simulink model "Winda4"  (R2016a)
settings: Solver=FixedStepDiscrete  StartTime=0.0  StopTime=inf  FixedStep=0.05  MaxStep=0.1  MinStep=0.01  RelTol=1e-3
libraries: simulink x15, realtime_pacer_lib x2
settings Model: Creator=dmar  LastModifiedBy=Kuba
settings DataIOCC: LimitDataPoints=on  SaveFormat=Array  SignalLoggingSaveFormat=ModelDataLogs  SignalLogging=off
settings OptimizationCC: BlockReduction=off  ConditionallyExecuteInputs=off  ExpressionDepthLimit=2147483647
settings DebuggingCC: AlgebraicLoopMsg=error  UnderspecifiedInitializationDetection=Classic  MergeDetectMultiDrivingBlocksExec=none  SolverPrmCheckMsg=warning  ParameterPrecisionLossMsg=none  FcnCallInpInsideContextMsg=UseLocalSettings  AllowSymbolicDim=off  StateNameClashWarn=warning
settings HardwareCC: ProdBitPerPointer=32  ProdLargestAtomicFloat=None  ProdIntDivRoundTo=Undefined  ProdEndianess=Unspecified  ProdWordSize=32  ProdHWDeviceType=ASIC/FPGA->ASIC/FPGA  ProdEqTarget=off
settings ModelReferenceCC: PropagateSignalLabelsOutOfModel=off
settings SFSimCC: SimParseCustomCode=off
settings GRTTargetCC: CombineOutputUpdateFcns=off  GRTInterface=on
settings ConfigComp: CovModelRefEnable=Off

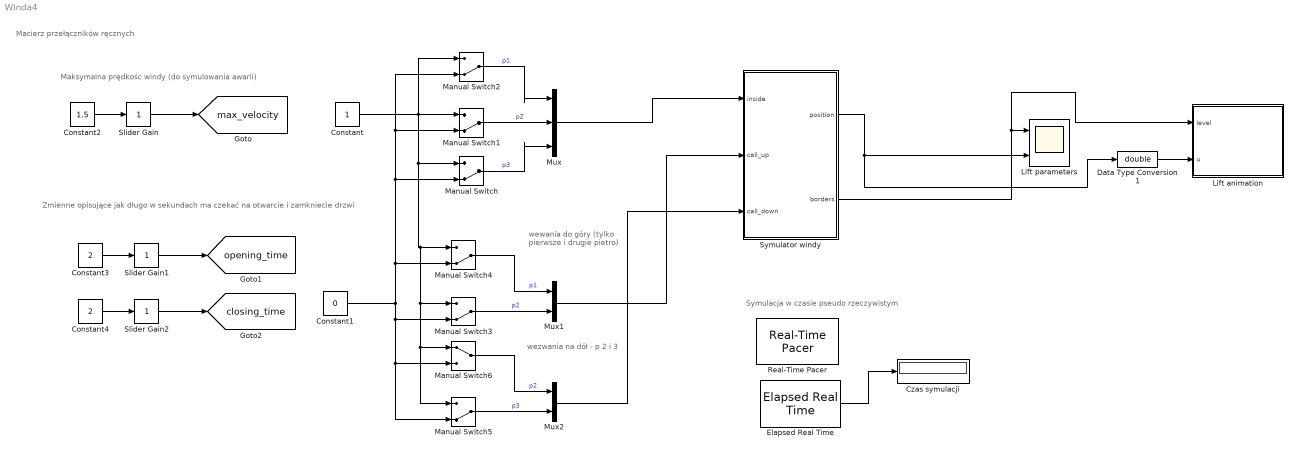
== system Winda4 ==
  note: wezwania na dół - p 2 i 3
  note: wewania do góry
      | (tylko pierwsze i drugie
      | pietro)
  note: Zmienne opisujące jak długo w sekundach ma czekać na otwarcie i zamkniecie drzwi
  note: Maksymalna prędkośc windy (do symulowania awarii)
  note: Macierz przełączników ręcznych
  note: Symulacja w czasie pseudo rzeczywistym
  Constant : Constant
  Constant1 : Constant  Value=0
  Constant2 : Constant  Value=1.5
  Constant3 : Constant  Value=2
  Constant4 : Constant  Value=2
  Czas symulacji : Display
  Data Type Conversion1 : DataTypeConversion  OutDataTypeStr=double
  Elapsed Real Time : realtime_pacer_lib/Elapsed Real Time
  Lift animation : MATLAB Function  TreatAsAtomicUnit=on  SystemSampleTime=0.05
  Lift parameters : Scope  NumInputPorts=2
  Manual Switch{,1..5} (6 alike) : ManualSwitch  CurrentSetting=0
  Manual Switch6 : ManualSwitch
  Mux : Mux  Inputs=3
  Mux1 : Mux  Inputs=2
  Mux2 : Mux  Inputs=2
  Real-Time Pacer : realtime_pacer_lib/Real-Time Pacer  simTimePerRealTime=1
  Slider Gain : simulink/Math Operations/Slider Gain  low=0  gain=1  high=1
  Slider Gain1 : simulink/Math Operations/Slider Gain  low=0  gain=1  high=1
  Slider Gain2 : simulink/Math Operations/Slider Gain  low=0  gain=1  high=1
  Symulator windy : Subsystem
  tag scope: closing_time=global, max_velocity=global, opening_time=global
  wires:
  Data Type Conversion1/1 -> Lift animation/2(u)
  Symulator windy/1(position) -> Data Type Conversion1/1, Lift parameters/2
  Symulator windy/2(borders) -> Lift animation/1(level), Lift parameters/1
  Elapsed Real Time/1 -> Czas symulacji/1
  Mux/1 -> Symulator windy/1(inside)
  Mux1/1 -> Symulator windy/2(call_up)
  Mux2/1 -> Symulator windy/3(call_down)
  Manual Switch6/1 -> Mux2/1  "p2"
  Constant/1 -> Manual Switch2/1, Manual Switch6/1, Manual Switch5/1, Manual Switch3/1, Manual Switch4/1, Manual Switch/1, Manual Switch1/1
  Constant1/1 -> Manual Switch2/2, Manual Switch1/2, Manual Switch/2, Manual Switch4/2, Manual Switch5/2, Manual Switch6/2, Manual Switch3/2
  Manual Switch5/1 -> Mux2/2  "p3"
  Manual Switch3/1 -> Mux1/2  "p2"
  Manual Switch4/1 -> Mux1/1  "p1"
  Manual Switch1/1 -> Mux/2  "p2"
  Manual Switch/1 -> Mux/3  "p3"
  Manual Switch2/1 -> Mux/1  "p1"
  Constant2/1 -> Slider Gain/1
  Slider Gain/1 -> [max_velocity]
  Constant3/1 -> Slider Gain1/1
  Slider Gain1/1 -> [opening_time]
  Constant4/1 -> Slider Gain2/1
  Slider Gain2/1 -> [closing_time]

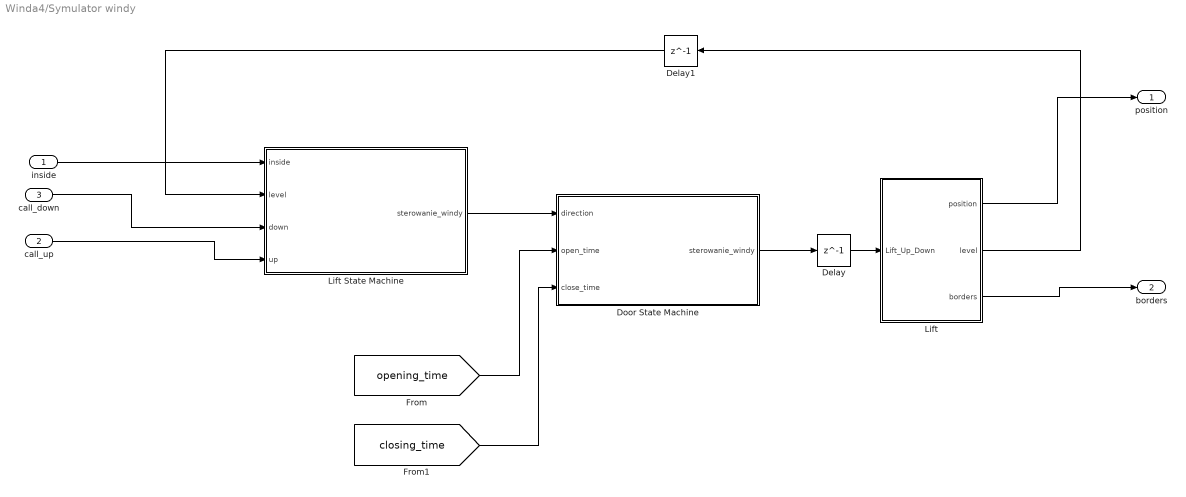
== system Winda4/Symulator windy ==
  inside : Inport
  call_up : Inport  Port=2
  call_down : Inport  Port=3
  Delay : Delay  DelayLength=1  InitialCondition=0
  Delay1 : Delay  DelayLength=1  InitialCondition=0
  Door State Machine : Stateflow chart  TreatAsAtomicUnit=on
  Lift : Subsystem
  Lift State Machine : Stateflow chart  TreatAsAtomicUnit=on
  position : Outport
  borders : Outport  Port=2
  wires:
  Lift/1(position) -> position/1
  Delay/1 -> Lift/1(Lift_Up_Down)
  inside/1 -> Lift State Machine/1(inside)
  Lift/2(level) -> Delay1/1
  Lift/3(borders) -> borders/1
  Delay1/1 -> Lift State Machine/2(level)
  Door State Machine/1(sterowanie_windy) -> Delay/1
  Lift State Machine/1(sterowanie_windy) -> Door State Machine/1(direction)
  call_down/1 -> Lift State Machine/3(down)
  call_up/1 -> Lift State Machine/4(up)
  [opening_time] -> Door State Machine/2(open_time)
  [closing_time] -> Door State Machine/3(close_time)

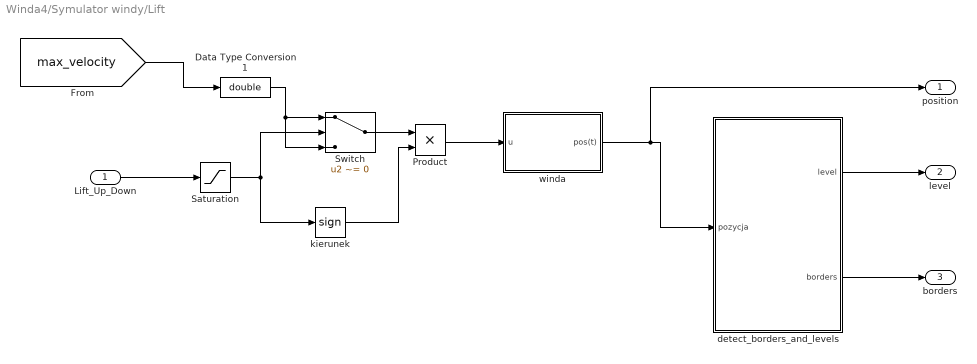
== system Winda4/Symulator windy/Lift ==
  Lift_Up_Down : Inport  OutDataTypeStr=int8
  Data Type Conversion1 : DataTypeConversion  OutDataTypeStr=double
  Product : Product  OutDataTypeStr=Inherit: Inherit via back propagation  RndMeth=Zero
  Saturation : Saturate  UpperLimit=1  LowerLimit=-1
  Switch : Switch  Criteria=u2 ~= 0  OutDataTypeStr=Inherit: Inherit via back propagation
  detect_borders_and_levels : Subsystem
  kierunek : Signum
  winda : Subsystem
  position : Outport
  level : Outport  Port=2
  borders : Outport  Port=3
  wires:
  Lift_Up_Down/1 -> Saturation/1
  Switch/1 -> Product/1
  Product/1 -> winda/1(u)
  kierunek/1 -> Product/2
  winda/1(pos(t)) -> detect_borders_and_levels/1(pozycja), position/1
  Saturation/1 -> Switch/2, kierunek/1
  detect_borders_and_levels/1(level) -> level/1
  detect_borders_and_levels/2(borders) -> borders/1
  [max_velocity] -> Data Type Conversion1/1
  Data Type Conversion1/1 -> Switch/3, Switch/1

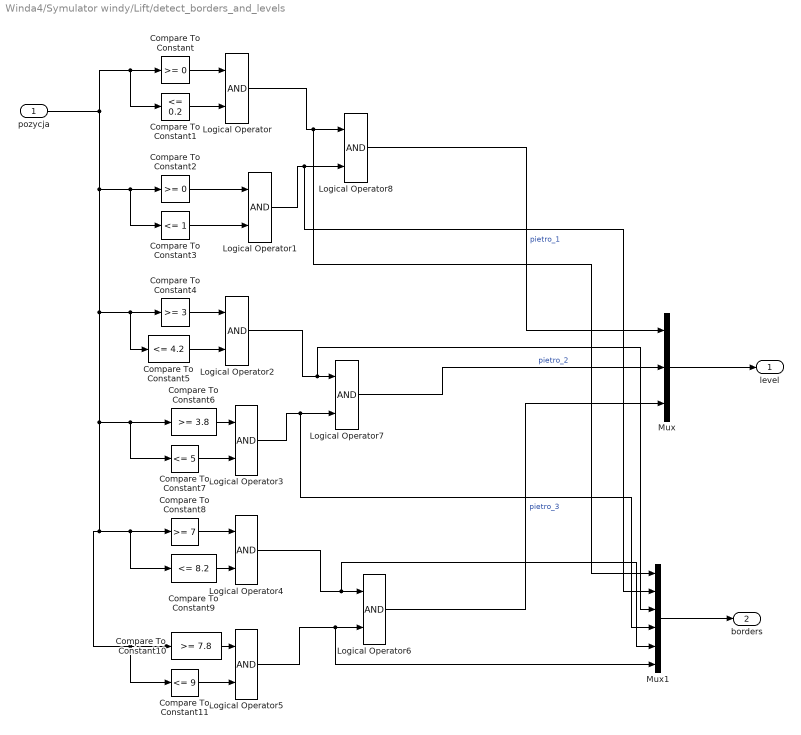
== system Winda4/Symulator windy/Lift/detect_borders_and_levels ==
  pozycja : Inport
  Compare To Constant : simulink/Logic and Bit Operations/Compare To Constant  relop=>=  const=0  OutDataTypeStr=boolean
  Compare To Constant1 : simulink/Logic and Bit Operations/Compare To Constant  relop=<=  const=0.2  OutDataTypeStr=boolean
  Compare To Constant10 : simulink/Logic and Bit Operations/Compare To Constant  relop=>=  const=7.8  OutDataTypeStr=boolean
  Compare To Constant11 : simulink/Logic and Bit Operations/Compare To Constant  relop=<=  const=9  OutDataTypeStr=boolean
  Compare To Constant2 : simulink/Logic and Bit Operations/Compare To Constant  relop=>=  const=0  OutDataTypeStr=boolean
  Compare To Constant3 : simulink/Logic and Bit Operations/Compare To Constant  relop=<=  const=1  OutDataTypeStr=boolean
  Compare To Constant4 : simulink/Logic and Bit Operations/Compare To Constant  relop=>=  const=3  OutDataTypeStr=boolean
  Compare To Constant5 : simulink/Logic and Bit Operations/Compare To Constant  relop=<=  const=4.2  OutDataTypeStr=boolean
  Compare To Constant6 : simulink/Logic and Bit Operations/Compare To Constant  relop=>=  const=3.8  OutDataTypeStr=boolean
  Compare To Constant7 : simulink/Logic and Bit Operations/Compare To Constant  relop=<=  const=5  OutDataTypeStr=boolean
  Compare To Constant8 : simulink/Logic and Bit Operations/Compare To Constant  relop=>=  const=7  OutDataTypeStr=boolean
  Compare To Constant9 : simulink/Logic and Bit Operations/Compare To Constant  relop=<=  const=8.2  OutDataTypeStr=boolean
  Logical Operator{,1..8} (9 alike) : Logic  AllPortsSameDT=off  OutDataTypeStr=boolean
  Mux : Mux  Inputs=3
  Mux1 : Mux  Inputs=6
  level : Outport
  borders : Outport  Port=2
  wires:
  Compare To Constant3/1 -> Logical Operator1/2
  Compare To Constant/1 -> Logical Operator/1
  Compare To Constant1/1 -> Logical Operator/2
  Compare To Constant4/1 -> Logical Operator2/1
  Compare To Constant2/1 -> Logical Operator1/1
  Compare To Constant10/1 -> Logical Operator5/1
  Compare To Constant11/1 -> Logical Operator5/2
  Compare To Constant8/1 -> Logical Operator4/1
  Compare To Constant7/1 -> Logical Operator3/2
  Compare To Constant6/1 -> Logical Operator3/1
  Compare To Constant9/1 -> Logical Operator4/2
  Compare To Constant5/1 -> Logical Operator2/2
  pozycja/1 -> Compare To Constant1/1, Compare To Constant/1, Compare To Constant10/1, Compare To Constant11/1, Compare To Constant9/1, Compare To Constant8/1, Compare To Constant6/1, Compare To Constant7/1, Compare To Constant5/1, Compare To Constant4/1, Compare To Constant2/1, Compare To Constant3/1
  Logical Operator4/1 -> Mux1/5, Logical Operator6/1
  Logical Operator5/1 -> Mux1/6, Logical Operator6/2
  Logical Operator1/1 -> Mux1/2, Logical Operator8/2
  Logical Operator/1 -> Mux1/1, Logical Operator8/1
  Logical Operator8/1 -> Mux/1  "pietro_1"
  Logical Operator2/1 -> Mux1/3, Logical Operator7/1
  Logical Operator3/1 -> Logical Operator7/2, Mux1/4
  Logical Operator7/1 -> Mux/2  "pietro_2"
  Logical Operator6/1 -> Mux/3  "pietro_3"
  Mux/1 -> level/1
  Mux1/1 -> borders/1

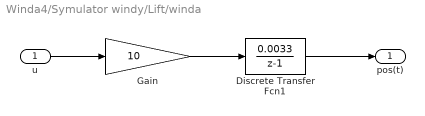
== system Winda4/Symulator windy/Lift/winda ==
  u : Inport  OutDataTypeStr=fixdt(1,26,12)
  Discrete Transfer Fcn1 : DiscreteTransferFcn  Numerator=[0.0033]  Denominator=[1 -1]  SampleTime=0.05  StateDataTypeStr=fixdt(1,26,12)  NumCoefDataTypeStr=fixdt(1,26,12)  DenCoefDataTypeStr=fixdt(1,26,12)  NumProductDataTypeStr=fixdt(1,26,12)  DenProductDataTypeStr=fixdt(1,26,12)  NumAccumDataTypeStr=fixdt(1,26,12)  DenAccumDataTypeStr=fixdt(1,26,12)  OutDataTypeStr=fixdt(1,26,12)
  Gain : Gain  Gain=10  ParamDataTypeStr=fixdt(1,15,2)  OutDataTypeStr=Inherit: Same as input
  pos(t) : Outport
  wires:
  Gain/1 -> Discrete Transfer Fcn1/1
  Discrete Transfer Fcn1/1 -> pos(t)/1
  u/1 -> Gain/1

== stateflow chart Winda4/Symulator windy/Lift State Machine ==
  settings: executeAtInitialization=1
  note: Maszyna stanów zarządzająca piętrami windy.
      | Uwzględnia wezwania
  state Pietro1
    entry: sterowanie_windy=0;
  state UP13
    entry: sterowanie_windy=1;
  state DOWN21
    entry: sterowanie_windy=-1;
  state UP12
    entry: sterowanie_windy=1;
  state Pietro2_DOWN
    entry: sterowanie_windy=0;
  state Pietro2
    entry: sterowanie_windy=0;
  state Pietro2_UP
    entry: sterowanie_windy=0;
  state UP23
    entry: sterowanie_windy=1;
  state DOWN32
    entry: sterowanie_windy=-1;
  state DOWN31
    entry: sterowanie_windy=-1;
  state Pietro3
    entry: sterowanie_windy=0;
  (default) -> Pietro1
  Pietro1 -> UP13 [order 2] : [inside[2]==1||down[1]==1]
  DOWN31 -> Pietro1 [order 1] : [level[0]==1]
  DOWN21 -> Pietro1 : [level[0]==1]
  Pietro1 -> UP12 [order 1] : [inside[1]==1||up[1]==1||down[0]==1]
  UP13 -> Pietro3 [order 1] : [level[2]==1]
  UP13 -> Pietro2_UP [order 2] : [level[1]==1&&up[1]==1]
  Pietro2_DOWN -> DOWN21 : [1]
  Pietro2 -> DOWN21 [order 1] : [inside[0]==1||up[0]==1]
  UP12 -> Pietro2 : [level[1]==1]
  DOWN32 -> Pietro2 : [level[1]==1]
  Pietro2 -> UP23 [order 2] : [inside[2]==1||down[1]==1]
  DOWN31 -> Pietro2_DOWN [order 2] : [level[1]==1&&down[1]==1]
  Pietro2_UP -> UP23 : [1]
  UP23 -> Pietro3 : [level[2]==1]
  Pietro3 -> DOWN32 [order 2] : [inside[1]==1||up[1]==1||down[0]==1]
  Pietro3 -> DOWN31 [order 1] : [inside[0]==1||up[0]==1]
  data: sterowanie_windy output int8; inside input; level input; down input; up input

== matlab function Winda4/Lift animation ==
  data: level input; u input
function plot_Lift3( level,u)
%#codegen




persistent fig3;
persistent NOWE1;
persistent L_pos;


if isempty(L_pos),

%     if isempty(fig3), 
%     fig3 = figure(3);
%     else
%     close(fig3);
%     fig3 = figure(3);
%     end
     %NOWE1 = [0 0.1 0.1 0 0; 0.25 .25 0 0 .25]*10;
    NOWE1 = [.1 0 0 .1 .1 .09 .09 .1; 0 0 0.25 0.25 0 0 0.12 .12]*10;
    
    axis([-4 4 -1 15]);
    grid('off');
    %xlabel('X position [m]');
    ylabel('Lift position [m]');
    hold('on');
    line([-0.05 -0.05],[0 12],'LineWidth',2,'Color','k')
    line([1.05 1.05],[0 12],'LineWidth',2,'Color','k')
    line([-4 4],[-0.05 -0.05],'LineWidth',2,'Color','k')
    
    line([-1 -0.05],[4 4],'LineWidth',2,'Color','k')
    line([1.05 2],[4 4],'LineWidth',2,'Color','k')
    
    line([-1 -0.05],[8 8],'LineWidth',2,'Color','k')
    line([1.05 2],[8 8],'LineWidth',2,'Color','k')
    
    line([-1 -0.05],[12 12],'LineWidth',2,'Color','k')
    line([1.05 2],[12 12],'LineWidth',2,'Color','k')
    
 % czarna lampka na wysokosci 0
 line([1.05 1.2],[0.2 0.2],'LineWidth',4,'Color','k')

 % czarna lampka na wysokosci 1
 line([1.05 1.2],[1 1],'LineWidth',4,'Color','k')
    
 % czarna lampka na wysokosci 4
 line([1.05 1.2],[4 4],'LineWidth',4,'Color','k')

 % czarna lampka na wysokosci 5
 line([1.05 1.2],[5 5],'LineWidth',4,'Color','k')
    
  % czarna lampka na wysokosci 8
 line([1.05 1.2],[8 8],'LineWidth',4,'Color','k')
 % czarna lampka na wysokosci 9
 line([1.05 1.2],[9 9],'LineWidth',4,'Color','k')
   
%plot(NOWE1(1,:),NOWE1(2,:)+prev1,'w');
L_pos=plot(NOWE1(1,:),NOWE1(2,:)+u,'b');
    
    
    
else
    if(ishghandle(L_pos)),
       
        set(L_pos,'yData',NOWE1(2,:)+u);


if level(1)==1    
 % czarna lampka na wysokosci 0
 line([1.05 1.2],[0.2 0.2],'LineWidth',4,'Color','r');
else
 line([1.05 1.2],[0.2 0.2],'LineWidth',4,'Color','k');
end

if level(2)==1    
 % czarna lampka na wysokosci 1
 line([1.05 1.2],[1 1],'LineWidth',4,'Color','r');
else
 line([1.05 1.2],[1 1],'LineWidth',4,'Color','k');
end

if level(3)==1    
 % czarna lampka na wysokosci 4
 line([1.05 1.2],[4 4],'LineWidth',4,'Color','r');
else
 line([1.05 1.2],[4 4],'LineWidth',4,'Color','k');
end

if level(4)==1    
 % czarna lampka na wysokosci 5
 line([1.05 1.2],[5 5],'LineWidth',4,'Color','r');
else
 line([1.05 1.2],[5 5],'LineWidth',4,'Color','k');
end

if level(5)==1    
 % czarna lampka na wysokosci 8
 line([1.05 1.2],[8 8],'LineWidth',4,'Color','r');
else
 line([1.05 1.2],[8 8],'LineWidth',4,'Color','k');
end

if level(6)==1    
 % czarna lampka na wysokosci 9
 line([1.05 1.2],[9 9],'LineWidth',4,'Color','r');
else
 line([1.05 1.2],[9 9],'LineWidth',4,'Color','k');
end



     
        
        
        
    end,
end

== stateflow chart Winda4/Symulator windy/Door State Machine ==
  settings: executeAtInitialization=1
  note: Maszyna stanów obsługi drzwi windy.
  state wait_for_call
    entry: sterowanie_windy=0;
    entry: timer=0;
  state close_door
    entry: sterowanie_windy=0;
    entry: timer = timer+0.05;
  state go
    entry: sterowanie_windy=direction;
    entry: timer=0;,
  state open_door
    entry: sterowanie_windy=0;
    entry: timer = timer+0.05;
  (default) -> wait_for_call
  open_door -> wait_for_call [order 1] : [timer>open_time]
  wait_for_call -> close_door : [direction ~= 0]
  close_door -> close_door [order 2] : [timer<close_time]
  close_door -> go [order 1] : [timer>close_time]
  go -> open_door : [direction == 0]
  open_door -> open_door [order 2] : [timer<close_time]
  data: sterowanie_windy output int8; direction input; open_time input; close_time input; timer local double
